simulink model "model"  (R2015a)
settings: Solver=ode45  StartTime=0.0  StopTime=10.0  RelTol=1e-3
libraries: PoliArd x6
settings Model: Creator=dell  LastModifiedBy=dell

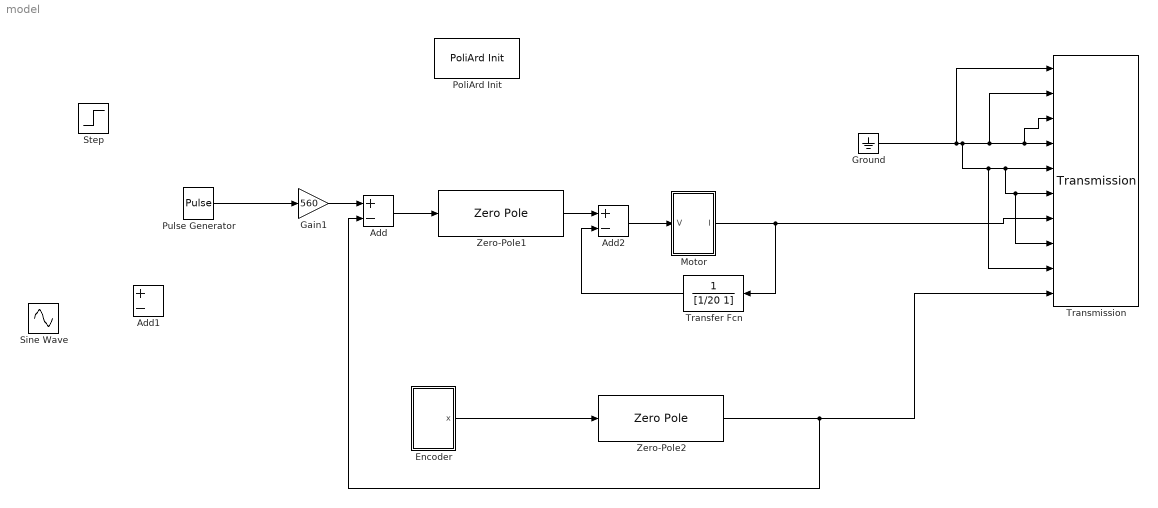
== system model ==
  Add : Sum  Inputs=+-
  Add1 : Sum  Inputs=+-
  Add2 : Sum  Inputs=+-
  "Encoder " : Subsystem
  Gain1 : Gain  Gain=560
  Ground : Ground
  Motor : Subsystem
  PoliArd Init : PoliArd/PoliArd Init
  Pulse Generator : DiscretePulseGenerator  PulseType=Time based  Amplitude=2  Period=10  PulseWidth=50  PhaseDelay=5
  Sine Wave : Sin  Amplitude=2  SampleTime=0
  Step : Step  SampleTime=0
  Transfer Fcn : TransferFcn  Denominator=[1/20 1]
  Transmission : PoliArd/Transmission  sample_freq=200  sig_to_send=6
  Zero-Pole1 : ZeroPole  Zeros=[]  Poles=[0,0]  Gain=-276.55
  Zero-Pole2 : ZeroPole  Zeros=[0]  Poles=[-100,-150]  Gain=1
  wires:
  Ground/1 -> Transmission/1, Transmission/9, Transmission/8, Transmission/6, Transmission/5, Transmission/2, Transmission/3, Transmission/4
  Gain1/1 -> Add/1
  Motor/1(I) -> Transfer Fcn/1, Transmission/7
  Add/1 -> Zero-Pole1/1
  Pulse Generator/1 -> Gain1/1
  Add2/1 -> Motor/1(V)
  Transfer Fcn/1 -> Add2/2
  "Encoder "/1(x) -> Zero-Pole2/1
  Zero-Pole2/1 -> Add/2, Transmission/10
  Zero-Pole1/1 -> Add2/1

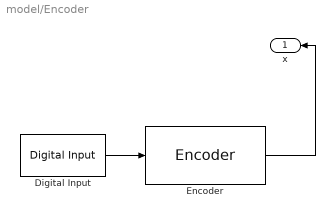
== system model/Encoder  ==
  Digital Input : PoliArd/Digital Input  DI_pin=2  DIsample=1/200
  Encoder : PoliArd/Encoder  EncoderID=1  dt_enc=-1
  x : Outport
  wires:
  Digital Input/1 -> Encoder/1
  Encoder/1 -> x/1

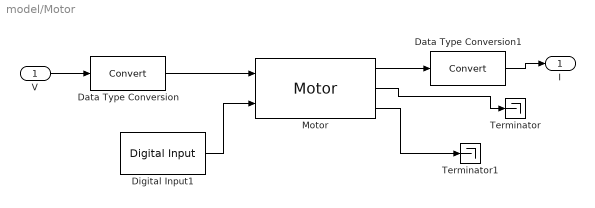
== system model/Motor ==
  V : Inport
  Data Type Conversion : DataTypeConversion
  Data Type Conversion1 : DataTypeConversion
  Digital Input1 : PoliArd/Digital Input  DI_pin=3  DIsample=1/200
  Motor : PoliArd/Motor  MotorID=1  DC_bus_mask=12  dt_mot=1/200
  Terminator : Terminator
  Terminator1 : Terminator
  I : Outport
  wires:
  Data Type Conversion/1 -> Motor/1
  Digital Input1/1 -> Motor/2
  V/1 -> Data Type Conversion/1
  Motor/3 -> Terminator1/1
  Motor/2 -> Terminator/1
  Motor/1 -> Data Type Conversion1/1
  Data Type Conversion1/1 -> I/1
